simulink model "BMS_V4"  (R2017b)
settings: Solver=FixedStepDiscrete  StartTime=0.0  StopTime=inf  FixedStep=BASETIME  RelTol=1e-3  EnableMultiTasking=on
values from neighbouring files (symbols this model uses):
  AKT_BALANCE = uint16(8)    [BMS_V4_config.m]
  BALANCE = uint16(4)    [BMS_V4_config.m]
  BALANCE_RESISTOR = int32(5)    [BMS_V4_config.m]
  BALANCE_VEC = uint16(8)    [BMS_V4_config.m]
  CELL_SOC = uint16(7)    [BMS_V4_config.m]
  CELL_STATE = uint16(3)    [BMS_V4_config.m]
  CELL_TEMPERATURE = uint16(6)    [BMS_V4_config.m]
  CELL_VOLTAGE = uint16(5)    [BMS_V4_config.m]
  CELLACTBITFIELD = hex2dec('300')    [BMS_V4_config.m]
  CELLDEACTBITFIELD = hex2dec('100')    [BMS_V4_config.m]
  CELLT_BURST = uint16(6)    [BMS_V4_config.m]
  CELLV_BURST = uint16(5)    [BMS_V4_config.m]
  CLK_CYC_timer_1 = 586    [BMS_V4_config.m]
  CLK_CYC_timer_2 = 5860    [BMS_V4_config.m]
  CLK_CYC_timer_3 = 280    [BMS_V4_config.m]
  CLK_CYC_timer_4 = 586*100    (= 58600)    [BMS_V4_config.m]
  CLK_CYC_timer_5 = 5800*2    (= 11600)    [BMS_V4_config.m]
  CLK_CYC_timer_6 = 320    [BMS_V4_config.m]
  CN_CELLS = int32(40*3600)    [BMS_V4_config.m]
  CONTACTOR = uint16(1)    [BMS_V4_config.m]
  CONTACTOR_LOCKED = uint16(0)    [BMS_V4_config.m]
  CONTACTOR_UNLOCKED = uint16(1)    [BMS_V4_config.m]
  DEBUG_SEND_STATES = uint16(hex2dec('01'))    [BMS_V4_config.m]
  DELTA_SOC_BALANCE = int32(5*1e6)    [BMS_V4_config.m]
  DELTA_SOC_BALANCE_OFF = int32(1*1e5)    [BMS_V4_config.m]
  DETERMINE_MODEL_PARAMETER_ACT = uint16(100)    [BMS_V4_config.m]
  DETERMINE_MODEL_PARAMETER_SCC = uint16(101)    [BMS_V4_config.m]
  ERROR = uint16(1)    [BMS_V4_config.m]
  EXTERN_SIGNALS = uint16(1)    [BMS_V4_config.m]
  FREQUENCY_STEPS = uint16([25 50 75 100 150 250 500 750                                      1000 1500 2500 5000 7500                                      10010 10015 10025 10050 10075                                      10100 10150 10250 10500 10750                                      11000 11500])    [BMS_V4_config.m]
  GET_IMAG_PART_MFC = uint16(9)    [BMS_V4_config.m]
  GET_IMAG_PART_MSF = uint16(4)    [BMS_V4_config.m]
  GET_REAL_PART_MFC = uint16(8)    [BMS_V4_config.m]
  GET_REAL_PART_MSF = uint16(3)    [BMS_V4_config.m]
  IMU = uint16(7)    [BMS_V4_config.m]
  IMU_AMP_OFF = uint16(5)    [BMS_V4_config.m]
  IMU_DATA_READ_LOCUS_ACT = uint16(6)    [BMS_V4_config.m]
  IMU_DATA_READ_LOCUS_SCC = uint16(7)    [BMS_V4_config.m]
  IMU_DEBUG = uint16(9)    [BMS_V4_config.m]
  IMU_GET_DATA_MFC = uint16(8)    [BMS_V4_config.m]
  IMU_GET_DATA_MSF = uint16(3)    [BMS_V4_config.m]
  IMU_OFFSET_POLLING = uint16(11)    [BMS_V4_config.m]
  IMU_POLLING = uint16(2)    [BMS_V4_config.m]
  IMU_POWER = uint16(10)    [BMS_V4_config.m]
  IMU_SEND_IMAG = uint16(11)    [BMS_V4_config.m]
  IMU_SEND_REAL = uint16(10)    [BMS_V4_config.m]
  INDEX_IMAGPART = uint16(2)    [BMS_V4_config.m]
  INDEX_REALPART = uint16(1)    [BMS_V4_config.m]
  INFO = uint16(2)    [BMS_V4_config.m]
  INIT_OFFSET_AMPLITUDE = uint16(2)    [BMS_V4_config.m]
  LINE_CURRENT = uint16(3)    [BMS_V4_config.m]
  LINE_CURRENT_CANA = uint16(4)    [BMS_V4_config.m]
  LINE_CURRENT_SWITCH_THRESHOLD = int32(2*1e6)    [BMS_V4_config.m]
  NUM_OF_CELLS = uint16(16)    [BMS_V4_config.m]
  NUM_OF_FREQUENCIES_PSO = uint16(14)    [BMS_V4_config.m]
  NUM_OF_LINES = uint16(1)    [BMS_V4_config.m]
  NUM_OF_PARAMETER = single(5)    [BMS_V4_config.m]
  NUM_OF_SOC_POINTS = uint16(110)    [BMS_V4_config.m]
  P_L_BOUND = single([0.05;0.01;0.1;0.01;0.1])    [BMS_V4_config.m]
  P_U_BOUND = single([0.50;0.20;0.9;0.06;60])    [BMS_V4_config.m]
  PARA_ACT_SEND = uint16(101)    [BMS_V4_config.m]
  PARA_DATA_STORE_ACT = uint16(8)    [BMS_V4_config.m]
  PARA_DATA_STORE_SCC = uint16(9)    [BMS_V4_config.m]
  PARA_SCC_SEND = uint16(102)    [BMS_V4_config.m]
  PARTICLE_INIT = single(create_startparticle(P_L_BOUND,P_U_BOUND,NUM_OF_PARTICLE))    [BMS_V4_config.m]
  POLACT = hex2dec('00000BFF')    [BMS_V4_config.m]
  POLDEACT = hex2dec('000008FF')    [BMS_V4_config.m]
  PSO_PARA_DEBUG = uint16(13)    [BMS_V4_config.m]
  REQUEST_SOC_REF = uint16(1000)    [BMS_V4_config.m]
  SCALE_FACTOR_CH1 = single(0.66666666)    [BMS_V4_config.m]
  SCALE_FACTOR_CH2 = single(0.66666666)    [BMS_V4_config.m]
  SEND_CELL_SOC_ABS = uint16(199)    [BMS_V4_config.m]
  SHUT_DOWN_BALANCE_OFF = uint16(3)    [BMS_V4_config.m]
  SHUT_DOWN_BALANCE_ON = uint16(2)    [BMS_V4_config.m]
  START_IMU_MSL = uint16(3)    [BMS_V4_config.m]
  START_IMU_SCC = uint16(1)    [BMS_V4_config.m]
  SWITCH_IMU_OFF = uint16(2)    [BMS_V4_config.m]
  SWITCH_IMU_ON = uint16(1)    [BMS_V4_config.m]
  SWITCH_IMU_ON_OFF = uint16(4)    [BMS_V4_config.m]
  SYSTEM_DEBUG = uint16(12)    [BMS_V4_config.m]
  TIMEOUT_CANA = uint32(5000)    [BMS_V4_config.m]
  TIMEOUT_GATEWAY = uint32(500)    [BMS_V4_config.m]
  TS_SOC = single(0.010)    [BMS_V4_config.m]
  WARNING = uint16(2)    [BMS_V4_config.m]
libraries: c280xlib x44, c2833xlib x5, simulink x2, c2000lib x1, idelinklib_common x1
(part 5 of 8)

== stateflow chart BMS_V4/MRAM_control ==
  state MRAM_send_command(mram_address,mram_data) [function]
  state Init
    en:
  state store_soc_CC
    state init
      en:
      cellNo_soc_cc=uint16(0);
      lineNo_soc_cc=uint16(0);
    state set_wren
      en:
      //write enable CODE 0x00
      MRAM_send_command(uint32(0),uint32(0));
    state Store_soc_CC
      en:
      mram_request=SOC_CC_STORE;
      MRAM_send_command(MRAM_soc_address(cellNo_soc_cc,SOC_CC_STORE),mram_convert_soc(cell_soc_CC[cellNo_soc_cc][lineNo_soc_cc]));
      // (cellNo_soc_cc,STORE_SOC_CC),MRAM_CONVERT_SOC(SoC_Cells_CC[cellNo_soc_cc],1)));
    state inc
      en:
      cellNo_soc_cc=cellNo_soc_cc+uint16(1);
    store_soc_CC.init -> store_soc_CC.set_wren
    store_soc_CC.set_wren -> store_soc_CC.Store_soc_CC : //after(0.0005,sec)
    (junction 64) -> store_soc_CC.set_wren
    (junction 63) -> (junction 64) [order 1] : [cellNo_soc_cc < NUM_OF_CELLS]
    store_soc_CC.Store_soc_CC -> store_soc_CC.inc : //after(0.01,sec)
        | [mram_value_read == true]
        | {mram_value_read = false;}
    store_soc_CC.inc -> (junction 63) : //after(0.0005,sec)
  state store_soc_ABS
    state init
      en:
      cellNo_soc_abs=uint16(0);
      lineNo_soc_abs=uint16(0);
    state set_wren
      en:
      //write enable CODE 0x00
      MRAM_send_command(uint32(0),uint32(0));
    state Store_soc_CC
      en:
      mram_request=SOC_ABS_STORE;
      MRAM_send_command(MRAM_soc_address(cellNo_soc_abs,SOC_ABS_STORE),mram_convert_soc(cell_soc_ABS));
      // (cellNo_soc_cc,STORE_SOC_CC),MRAM_CONVERT_SOC(SoC_Cells_CC[cellNo_soc_cc],1)));
    state inc
      en:
    store_soc_ABS.init -> store_soc_ABS.set_wren
    store_soc_ABS.set_wren -> store_soc_ABS.Store_soc_CC : //after(0.0005,sec)
    store_soc_ABS.Store_soc_CC -> store_soc_ABS.inc : //after(0.01,sec)
        | [mram_value_read == true]
        | {mram_value_read = false;}
  state read_soc_CC
    state init
      en:
      cellNo_soc_cc=uint16(0);
      lineNo_soc_cc=uint16(0);
    state Store_soc_CC
      en:
      mram_value_read = false;
      mram_request=SOC_CC_READ;
      MRAM_send_command(MRAM_soc_address(cellNo_soc_cc,SOC_CC_READ),uint32(0));
      // (cellNo_soc_cc,STORE_SOC_CC),MRAM_CONVERT_SOC(SoC_Cells_CC[cellNo_soc_cc],1)));
    state inc
      en:
      cell_soc_CC[cellNo_soc_cc][lineNo_soc_cc] = mram_convert_unit32_to_int32(spi_rx_msg);
      cellNo_soc_cc=cellNo_soc_cc+uint16(1);
    read_soc_CC.init -> read_soc_CC.Store_soc_CC
    (junction 83) -> read_soc_CC.Store_soc_CC [order 1] : [cellNo_soc_cc < NUM_OF_CELLS]
    read_soc_CC.Store_soc_CC -> read_soc_CC.inc : [mram_value_read == true]
    read_soc_CC.inc -> (junction 83) : //after(0.0005,sec)
  state read_soc_ABS
    state init
      en:
      cellNo_soc_abs=uint16(0);
      lineNo_soc_abs=uint16(0);
    state Store_soc_CC
      en:
      mram_value_read = false;
      mram_request=SOC_ABS_READ;
      MRAM_send_command(MRAM_soc_address(cellNo_soc_abs,SOC_ABS_READ),uint32(0));
      // (cellNo_soc_cc,STORE_SOC_CC),MRAM_CONVERT_SOC(SoC_Cells_CC[cellNo_soc_cc],1)));
    state inc
      en:
      cell_soc_ABS = mram_convert_unit32_to_int32(spi_rx_msg);
    read_soc_ABS.init -> read_soc_ABS.Store_soc_CC
    read_soc_ABS.Store_soc_CC -> read_soc_ABS.inc : [mram_value_read == true]
  state store_imu_data
    state store_imu_data_actual
      state init
        en:
        cellNo_store_imu=uint16(imu_act_cellno-uint16(1));
        lineNo_store_imu=uint16(0);
        soc_store_imu=imu_act_soc;
        freq_ind_store_imu=uint16(imu_act_freq_index-uint16(1));
        store_realpart = mram_convert_single_to_uint32(imu_act_realpart);
        store_imagpart = mram_convert_single_to_uint32(imu_act_imagpart);
        mram_value_stored = false;
      state set_wren
        en:
        //write enable CODE 0x00
        MRAM_send_command(uint32(0),uint32(0));
      state Store_imu_data_soc
        en:
        //mram_value_stored = false;
        mram_request=IMU_DATA_STORE_SOC_POINT;
        MRAM_send_command(MRAM_soc_address(cellNo_store_imu,IMU_DATA_STORE_SOC_POINT),mram_convert_soc(soc_store_imu));
      state set_wren1
        en:
        //write enable CODE 0x00
        MRAM_send_command(uint32(0),uint32(0));
      state Store_imu_data_realpart
        en:
        mram_request=IMU_DATA_STORE_REAL;
        store_address = MRAM_imu_data_address_actual(cellNo_store_imu,freq_ind_store_imu,IMU_DATA_STORE_REAL);
        MRAM_send_command(store_address,store_realpart);
      state set_wren2
        en:
        //write enable CODE 0x00
        MRAM_send_command(uint32(0),uint32(0));
      state Store_imu_data_imagpart
        en:
        mram_request=IMU_DATA_STORE_IMAG;
        store_address = MRAM_imu_data_address_actual(cellNo_store_imu,freq_ind_store_imu,IMU_DATA_STORE_IMAG);
        MRAM_send_command(store_address,store_imagpart);
      store_imu_data.store_imu_data_actual.init -> store_imu_data.store_imu_data_actual.set_wren
      store_imu_data.store_imu_data_actual.set_wren -> Store_imu_data_soc : [mram_value_stored == true]
          | {mram_value_stored = false;}
      Store_imu_data_soc -> set_wren1 : [mram_value_stored == true]
          | {mram_value_stored = false;}
      set_wren1 -> store_imu_data.store_imu_data_actual.Store_imu_data_realpart : //after(0.0005,sec)
          | [mram_value_stored == true]
          | {mram_value_stored = false;}
      store_imu_data.store_imu_data_actual.Store_imu_data_realpart -> store_imu_data.store_imu_data_actual.set_wren2 : [mram_value_stored == true]
          | {mram_value_stored = false;}
      store_imu_data.store_imu_data_actual.set_wren2 -> store_imu_data.store_imu_data_actual.Store_imu_data_imagpart : //after(0.0005,sec)
          | [mram_value_stored == true]
          | {mram_value_stored = false;}
    state store_imu_data_scc
      state init
        en:
        cellNo_store_imu=uint16(imu_act_cellno-uint16(1));
        lineNo_store_imu=uint16(0);
        //convert soc to 0, 1, 2, ..., 98, 99,100% for mram adress config
        soc_point_store = soc_point_counter;
        freq_ind_store_imu=uint16(imu_act_freq_index-uint16(1));
        store_realpart = mram_convert_single_to_uint32(imu_act_realpart);
        store_imagpart = mram_convert_single_to_uint32(imu_act_imagpart);
        mram_value_stored = false;
      state set_wren
        en:
        //write enable CODE 0x00
        MRAM_send_command(uint32(0),uint32(0));
      state Store_imu_data_realpart
        en:
        //mram_value_stored = false;
        mram_request=IMU_DATA_STORE_REAL;
        store_address = MRAM_imu_data_address(cellNo_store_imu,soc_point_store,freq_ind_store_imu,IMU_DATA_STORE_REAL);
        MRAM_send_command(store_address,store_realpart);
      state set_wren2
        en:
        //write enable CODE 0x00
        MRAM_send_command(uint32(0),uint32(0));
      state Store_imu_data_imagpart
        en:
        mram_request=IMU_DATA_STORE_IMAG;
        store_address = MRAM_imu_data_address(cellNo_store_imu,soc_point_store,freq_ind_store_imu,IMU_DATA_STORE_IMAG);
        MRAM_send_command(store_address,store_imagpart);
      store_imu_data.store_imu_data_scc.init -> store_imu_data.store_imu_data_scc.set_wren
      store_imu_data.store_imu_data_scc.set_wren -> store_imu_data.store_imu_data_scc.Store_imu_data_realpart : [mram_value_stored == true]
          | {mram_value_stored = false;}
      store_imu_data.store_imu_data_scc.Store_imu_data_realpart -> store_imu_data.store_imu_data_scc.set_wren2 : [mram_value_stored == true]
          | {mram_value_stored = false;}
      store_imu_data.store_imu_data_scc.set_wren2 -> store_imu_data.store_imu_data_scc.Store_imu_data_imagpart : [mram_value_stored == true]
          | {mram_value_stored = false;}
    (junction 230) -> store_imu_data.store_imu_data_scc.init [order 1] : [imu_function == START_IMU_SCC]
    (junction 230) -> store_imu_data.store_imu_data_actual.init [order 2] : [ imu_function == START_IMU_MSL ]
    store_imu_data.store_imu_data_scc.Store_imu_data_imagpart -> (junction 236) : [mram_value_stored == true]
        | {mram_value_stored = false;}
    store_imu_data.store_imu_data_actual.Store_imu_data_imagpart -> (junction 236) : [mram_value_stored == true]
        | {mram_value_stored = false;}
  state read_imu_data_act
    state read_soc_point_imu_data
      en:
      cellNo_read_locus=mram_cellno_to_read-uint16(1);
      mram_request=IMU_DATA_READ_SOC_POINT;
      MRAM_send_command(MRAM_soc_address(cellNo_read_locus,IMU_DATA_READ_SOC_POINT),uint32(0));
    state store_soc_point_imu_data
      en:
      soc_of_one_locus_act = mram_convert_unit32_to_int32(spi_rx_msg);
      freq_ind_read_locus=uint16(0);
    state read_realpart_imu_data
      en:
      mram_request=IMU_DATA_READ_REAL;
      MRAM_send_command(MRAM_imu_data_address_actual(cellNo_read_locus,freq_ind_read_locus,IMU_DATA_READ_REAL),uint32(0));
    state store_real_part_and_read_imagpart_imu_data
      en:
      one_locus_act[freq_ind_read_locus][uint16(0)] = mram_convert_uint32_to_single(spi_rx_msg);
      mram_request=IMU_DATA_READ_IMAG;
      MRAM_send_command(MRAM_imu_data_address_actual(cellNo_read_locus,freq_ind_read_locus,IMU_DATA_READ_IMAG),uint32(0));
    state store_imag_part
      en:
      one_locus_act[freq_ind_read_locus][uint16(1)] = mram_convert_uint32_to_single(spi_rx_msg);
    read_soc_point_imu_data -> read_imu_data_act.store_soc_point_imu_data : //after(0.01,sec)
        | [mram_value_read == true]
        | {mram_value_read = false;}
    read_imu_data_act.store_soc_point_imu_data -> read_imu_data_act.read_realpart_imu_data : //after(0.01,sec)
        | //[mram_value_read == true]
        | //{mram_value_read = false;}
    (junction 894) -> read_imu_data_act.read_realpart_imu_data
    (junction 893) -> (junction 894)
    read_imu_data_act.read_realpart_imu_data -> store_real_part_and_read_imagpart_imu_data : //after(0.01,sec)
        | [mram_value_read == true]
        | {mram_value_read = false;}
    store_real_part_and_read_imagpart_imu_data -> read_imu_data_act.store_imag_part : //after(0.01,sec)
        | [mram_value_read == true]
        | {mram_value_read = false;}
    read_imu_data_act.store_imag_part -> (junction 893) [order 1] : [freq_ind_read_locus < (NUM_OF_FREQUENCIES-uint16(1))]
        | {freq_ind_read_locus++;}
  state read_imu_data_scc
    state init
      en:
      cellNo_read_locus = mram_cellno_to_read-uint16(1);
      socpoint_read_locus = mram_soc_point_to_read - uint16(1);
      freq_ind_read_locus=uint16(0);
    state read_realpart_imu_data
      en:
      mram_request=IMU_DATA_READ_REAL;
      MRAM_send_command(MRAM_imu_data_address(cellNo_read_locus,socpoint_read_locus,freq_ind_read_locus,IMU_DATA_READ_REAL),uint32(0));
    state store_real_part_and_read_imagpart_imu_data1
      en:
      one_locus_scc[freq_ind_read_locus][uint16(0)] = mram_convert_uint32_to_single(spi_rx_msg);
      mram_request=IMU_DATA_READ_IMAG;
      MRAM_send_command(MRAM_imu_data_address(cellNo_read_locus,socpoint_read_locus,freq_ind_read_locus,IMU_DATA_READ_IMAG),uint32(0));
    state store_imag_part
      en:
      one_locus_scc[freq_ind_read_locus][uint16(1)] = mram_convert_uint32_to_single(spi_rx_msg);
    read_imu_data_scc.init -> read_imu_data_scc.read_realpart_imu_data : after(0.0005,sec)
    (junction 871) -> read_imu_data_scc.read_realpart_imu_data
    (junction 875) -> (junction 871)
    read_imu_data_scc.read_realpart_imu_data -> store_real_part_and_read_imagpart_imu_data1 : //after(0.01,sec)
        | [mram_value_read == true]
        | {mram_value_read = false;}
    store_real_part_and_read_imagpart_imu_data1 -> read_imu_data_scc.store_imag_part : //after(0.01,sec)
        | [mram_value_read == true]
        | {mram_value_read = false;}
    read_imu_data_scc.store_imag_part -> (junction 875) [order 1] : [freq_ind_read_locus < (NUM_OF_FREQUENCIES-uint16(1))]
        | {freq_ind_read_locus++;}
  state store_para_data_act
    //stores all 6 parameter
    // of one cell
    state init
      en:
      num_para_store = uint16(0);
      cellNo_store_para=uint16(para_act_cellno-uint16(1));
      lineNo_store_para=uint16(0);
    state select_parameter
      en:
      store_parameter = mram_convert_single_to_uint32(parameter_one_cell_act[num_para_store]);
    state set_wren
      en:
      //write enable CODE 0x00
      MRAM_send_command(uint32(0),uint32(0));
    state Store_para_data
      en:
      //mram_value_stored = false;
      mram_request=PARA_STORE_ACT;
      store_address = MRAM_para_address_act(cellNo_store_para,num_para_store, PARA_STORE_ACT);
      MRAM_send_command(store_address,store_parameter);
    store_para_data_act.init -> store_para_data_act.select_parameter
    (junction 659) -> store_para_data_act.select_parameter
    (junction 657) -> (junction 659) [order 1] : [num_para_store < NUM_OF_PARAMETER]
        | {num_para_store++;}
        | // num of parameter = 5, but here we save 6 parameter
        | // parameter 6 is L2norm
    store_para_data_act.select_parameter -> store_para_data_act.set_wren
    (junction 745) -> (junction 746)
    store_para_data_act.set_wren -> store_para_data_act.Store_para_data : [mram_value_stored == true]
        | {mram_value_stored = false;}
    store_para_data_act.Store_para_data -> (junction 657) : [mram_value_stored == true]
        | {mram_value_stored = false;}
    (junction 657) -> (junction 744) [order 2]
    (junction 744) -> (junction 745)
  state store_para_data_scc
    //stores all  parameter of scc  0% SoC -> 100%SoC
    //of one cell
    state init
      en:
      num_para_store = uint16(0);
      cellNo_store_para = para_act_cellno-uint16(1);
      lineNo_store_para = uint16(0);
      soc_point_store_scc = uint16(0); // 0 indexing in simulink 1-101 for 0% - 100%
    state select_parameter
      en:
      store_parameter = mram_convert_single_to_uint32(parameter_one_cell_scc[soc_point_store_scc][num_para_store]);
      store_address = MRAM_para_address_scc(cellNo_store_para,num_para_store,soc_point_store_scc, PARA_STORE_SCC);
    state set_wren
      en:
      //write enable CODE 0x00
      MRAM_send_command(uint32(0),uint32(0));
    state Store_para_data
      en:
      //mram_value_stored = false;
      mram_request=PARA_STORE_SCC;
      MRAM_send_command(store_address,store_parameter);
    store_para_data_scc.init -> store_para_data_scc.select_parameter
    (junction 924) -> store_para_data_scc.select_parameter [order 1] : //[soc_point_store_scc < (NUM_OF_SOC_POINTS-uint16(1))]
        | [soc_point_store_scc < (last_soc_point_index - uint16(1))]
        | {soc_point_store_scc ++;}
    (junction 912) -> (junction 924)
    (junction 923) -> store_para_data_scc.select_parameter
    (junction 926) -> (junction 923) [order 1] : [num_para_store < NUM_OF_PARAMETER]
        | {num_para_store++;}
        | // num of parameter = 5, but here we save 6 parameter
        | // parameter 6 is L2norm
    store_para_data_scc.select_parameter -> store_para_data_scc.set_wren
    store_para_data_scc.set_wren -> store_para_data_scc.Store_para_data : [mram_value_stored == true]
        | {mram_value_stored = false;}
    store_para_data_scc.Store_para_data -> (junction 926) : [mram_value_stored == true]
        | {mram_value_stored = false;}
    (junction 926) -> (junction 925) [order 2] : {num_para_store = uint16(0);}
    (junction 925) -> (junction 912)
  state read_para_data_act
    // read parameter set from last impedance measurement of one cell.
    // global variable parameterset_one_cell coresponding soc is stored at soc adress from actual imu
    state read_soc_point_para_data
      en:
      num_para_read = uint16(0);
      cellNo_read_para=para_act_cellno-uint16(1);
      mram_request=IMU_DATA_READ_SOC_POINT;
      MRAM_send_command(MRAM_soc_address(cellNo_read_para,IMU_DATA_READ_SOC_POINT),uint32(0));
    state store_soc_point_imu_data
      en:
      soc_of_one_para_act = mram_convert_unit32_to_int32(spi_rx_msg); // same soc of locus meas act
      //soc_of_one_locus_act = mram_convert_unit32_to_int32(spi_rx_msg);
    state Read_para_data
      en:
      //mram_value_stored = false;
      mram_request=PARA_READ_ACT;
      MRAM_send_command(MRAM_para_address_act(cellNo_read_para,num_para_read, PARA_READ_ACT),uint32(0));
    state save_para_data
      en:
      parameter_one_cell_act[num_para_read] = mram_convert_uint32_to_single(spi_rx_msg);
    read_soc_point_para_data -> read_para_data_act.store_soc_point_imu_data : //after(0.01,sec)
        | [mram_value_read == true]
        | {mram_value_read = false;}
    read_para_data_act.store_soc_point_imu_data -> read_para_data_act.Read_para_data : //after(0.01,sec)
        | //[mram_value_read == true]
        | //{mram_value_read = false;}
    (junction 1036) -> read_para_data_act.Read_para_data
    (junction 1029) -> (junction 1036) [order 1] : [num_para_read < NUM_OF_PARAMETER]
        | {num_para_read++;}
        | // num of parameter = 5, but here we save 6 parameter
        | // parameter 6 is L2norm
    read_para_data_act.Read_para_data -> read_para_data_act.save_para_data : //after(0.01,sec)
        | [mram_value_read == true]
        | {mram_value_read = false;}
    (junction 1031) -> (junction 1035)
    read_para_data_act.save_para_data -> (junction 1029)
    (junction 1029) -> (junction 1030) [order 2]
    (junction 1030) -> (junction 1031)
  state read_para_data_scc
    // read parameter set from last impedance measurement of one cell.
    // global variable parameterset_one_cell coresponding soc is stored at soc adress from actual imu
    state init
      en:
      num_para_read = uint16(0);
      cellNo_read_para=para_act_cellno-uint16(1);
      soc_point_read_scc = uint16(0); // 0 indexing in simulink 1-101 for 0% - 100%
    state Read_para_data
      en:
      //mram_value_stored = false;
      mram_request=PARA_READ_SCC;
      MRAM_send_command(MRAM_para_address_scc(cellNo_read_para,num_para_read,soc_point_read_scc, PARA_READ_SCC),uint32(0));
    state save_para_data
      en:
      parameter_one_cell_scc[soc_point_read_scc][num_para_read] = mram_convert_uint32_to_single(spi_rx_msg);
    read_para_data_scc.init -> read_para_data_scc.Read_para_data
    (junction 1042) -> read_para_data_scc.Read_para_data [order 1] : //[soc_point_read_scc < (NUM_OF_SOC_POINTS-uint16(1))]
        | [soc_point_read_scc < (last_soc_point_index - uint16(1))]
        | {soc_point_read_scc ++;}
    (junction 1041) -> read_para_data_scc.Read_para_data
    (junction 1044) -> (junction 1042)
    (junction 1043) -> (junction 1041) [order 1] : [num_para_read < NUM_OF_PARAMETER]
        | {num_para_read++;}
        | // num of parameter = 5, but here we save 6 parameter
        | // parameter 6 is L2norm
    read_para_data_scc.Read_para_data -> read_para_data_scc.save_para_data : //after(0.01,sec)
        | [mram_value_read == true]
        | {mram_value_read = false;}
    read_para_data_scc.save_para_data -> (junction 1043) : //after(0.01,sec)
    (junction 1043) -> (junction 1045) [order 2] : {num_para_read = uint16(0);}
    (junction 1045) -> (junction 1044)
  state store_soc_SCC
    state init
      en:
      soc_point_scc = uint16(0);
    state set_wren
      en:
      //write enable CODE 0x00
      MRAM_send_command(uint32(0),uint32(0));
    state Store_soc_SCC
      en:
      mram_request=SOC_SCC_STORE;
      MRAM_send_command(MRAM_soc_scc_address(soc_point_scc,SOC_SCC_STORE),mram_convert_soc(soc_points_of_scc[soc_point_scc]));
      // (cellNo_soc_cc,STORE_SOC_CC),MRAM_CONVERT_SOC(SoC_Cells_CC[cellNo_soc_cc],1)));
    state inc
      en:
      soc_point_scc=soc_point_scc+uint16(1);
    store_soc_SCC.init -> store_soc_SCC.set_wren
    store_soc_SCC.set_wren -> Store_soc_SCC : //after(0.0005,sec)
    (junction 943) -> store_soc_SCC.set_wren
    (junction 944) -> (junction 943) [order 1] : //[soc_point_scc < NUM_OF_SOC_POINTS]
        | [soc_point_scc < last_soc_point_index]
    Store_soc_SCC -> store_soc_SCC.inc : //after(0.01,sec)
        | [mram_value_read == true]
        | {mram_value_read = false;}
    store_soc_SCC.inc -> (junction 944) : //after(0.0005,sec)
  state read_soc_SCC
    state init
      en:
      soc_point_scc = uint16(0);
    state set_wren
      en:
      //write enable CODE 0x00
      MRAM_send_command(uint32(0),uint32(0));
    state Read_soc_SCC
      en:
      mram_request=SOC_SCC_READ;
      MRAM_send_command(MRAM_soc_scc_address(soc_point_scc,SOC_SCC_READ),uint32(0));
    state store_value_and_inc
      en:
      soc_points_of_scc[soc_point_scc] = mram_convert_unit32_to_int32(spi_rx_msg);
      soc_point_scc=soc_point_scc+uint16(1);
    read_soc_SCC.init -> read_soc_SCC.set_wren
    read_soc_SCC.set_wren -> Read_soc_SCC : //after(0.0005,sec)
    (junction 974) -> read_soc_SCC.set_wren
    (junction 975) -> (junction 974) [order 1] : //[soc_point_scc < NUM_OF_SOC_POINTS]
        | [soc_point_scc < last_soc_point_index]
    Read_soc_SCC -> store_value_and_inc : //after(0.01,sec)
        | [mram_value_read == true]
        | {mram_value_read = false;}
    store_value_and_inc -> (junction 975) : //after(0.0005,sec)
  state store_last_soc_index
    state set_wren
      en:
      //write enable CODE 0x00
      MRAM_send_command(uint32(0),uint32(0));
    state Store_soc_CC
      en:
      MRAM_send_command(MRAM_address_scc_soc_index(STORE_LAST_SOC_INDEX),uint32(last_soc_point_index));
    state wait_
      en:
    store_last_soc_index.set_wren -> store_last_soc_index.Store_soc_CC : //after(0.0005,sec)
    store_last_soc_index.Store_soc_CC -> wait_ : //after(0.01,sec)
        | [mram_value_read == true]
        | {mram_value_read = false;}
  state read_last_soc_index
    state Store_soc_CC
      en:
      MRAM_send_command(MRAM_address_scc_soc_index(READ_LAST_SOC_INDEX),uint32(0));
    state save
      en:
      last_soc_point_index = uint16(spi_rx_msg);
    read_last_soc_index.Store_soc_CC -> save : //after(0.01,sec)
        | [mram_value_read == true]
        | {mram_value_read = false;}
  (junction 1090) -> store_last_soc_index.set_wren [order 1] : [ mram_command...
      | [STORE_LAST_SOC_INDEX_SCC - uint16(1)]...
      |  == true ]
  (junction 1111) -> read_last_soc_index.Store_soc_CC : [ mram_command...
      | [READ_LAST_SOC_INDEX_SCC - uint16(1)]...
      |  == true ]
  (junction 1035) -> (junction 560) : {mram_command...
      | [PARA_DATA_READ_ACT-uint16(1)]...
      | = false;}
  (junction 1042) -> (junction 638) [order 2] : {mram_command...
      | [PARA_DATA_READ_SCC-uint16(1)]...
      | = false;}
  (junction 989) -> read_soc_SCC.init [order 1] : [ mram_command...
      | [SOC_SCC_READ - uint16(1)]...
      |  == true ]
  (junction 958) -> store_soc_SCC.init [order 1] : [ mram_command...
      | [SOC_SCC_STORE - uint16(1)]...
      |  == true ]
  read_imu_data_scc.store_imag_part -> (junction 851) [order 2] : {mram_command...
      | [IMU_DATA_READ_LOCUS_SCC-uint16(1)]...
      | = false;}
  read_imu_data_act.store_imag_part -> (junction 178) [order 2] : {mram_command...
      | [IMU_DATA_READ_LOCUS_ACT-uint16(1)]...
      | = false;}
  (junction 849) -> read_imu_data_scc.init [order 1] : [ mram_command...
      | [IMU_DATA_READ_LOCUS_SCC-uint16(1)]...
      |  == true ]
  (junction 746) -> (junction 451) : {mram_command...
      | [PARA_DATA_STORE_ACT-uint16(1)]...
      | = false;}
  (junction 63) -> (junction 31) [order 2] : {mram_command...
      | [SOC_CC_STORE-uint16(1)]...
      | = false;}
  (junction 83) -> (junction 100) [order 2] : {mram_command...
      | [SOC_CC_READ-uint16(1)]...
      | = false;}
  (junction 21) -> store_soc_ABS.init [order 1] : [ mram_command...
      | [SOC_ABS_STORE-uint16(1)] ...
      | ==true ]
  (junction 728) -> read_soc_ABS.init [order 1] : [ mram_command...
      | [SOC_ABS_READ-uint16(1)]...
      |  == true ]
  read_soc_ABS.inc -> (junction 730) : {mram_command...
      | [SOC_ABS_READ-uint16(1)]...
      | = false;}
  (junction 975) -> (junction 990) [order 2] : {mram_command...
      | [SOC_SCC_READ-uint16(1)]...
      | = false;}
  (junction 944) -> (junction 962) [order 2] : {mram_command...
      | [SOC_SCC_STORE-uint16(1)]...
      | = false;}
  wait_ -> (junction 1094) : {mram_command...
      | [STORE_LAST_SOC_INDEX_SCC-uint16(1)]...
      | = false;}
  save -> (junction 1115) : {mram_command...
      | [READ_LAST_SOC_INDEX_SCC-uint16(1)]...
      | = false;}
  (junction 181) -> read_soc_point_imu_data [order 1] : [ mram_command...
      | [IMU_DATA_READ_LOCUS_ACT-uint16(1)]...
      |  == true ]
  (default) -> Init
  Init -> (junction 4) : [ (mram_command[0] || ...
      |    mram_command[1] || ...
      |    mram_command[2] || ...
      |    mram_command[3] || ...
      |    mram_command[4] || ...
      |    mram_command[5] || ...
      |    mram_command[6] || ...
      |    mram_command[7] || ...
      |    mram_command[8] || ...
      |    mram_command[9] || ...
      |    mram_command[10] || ...
      |    mram_command[11] || ...
      |    mram_command[12] || ...
      |    mram_command[13] || ...
      |    mram_command[14]) != 0]
  (junction 4) -> (junction 19)
  (junction 31) -> Init
  (junction 924) -> (junction 631) [order 2] : {mram_command...
      | [PARA_DATA_STORE_SCC-uint16(1)]...
      | = false;}
  (junction 236) -> (junction 120) : {mram_command...
      | [IMU_DATA_STORE-uint16(1)]...
      | = false;}
  (junction 19) -> store_soc_CC.init [order 1] : [ mram_command...
      | [SOC_CC_STORE-uint16(1)]...
      |  == true ]
  (junction 33) -> (junction 31)
  (junction 19) -> (junction 21) [order 2]
  store_soc_ABS.inc -> (junction 33) : {mram_command...
      | [SOC_ABS_STORE-uint16(1)]...
      | = false;}
  (junction 100) -> (junction 33)
  (junction 21) -> (junction 97) [order 2]
  (junction 730) -> (junction 100)
  (junction 97) -> (junction 728) [order 2]
  (junction 97) -> read_soc_CC.init [order 1] : [ mram_command...
      | [SOC_CC_READ-uint16(1)]...
      |  == true ]
  (junction 120) -> (junction 730)
  (junction 728) -> (junction 123) [order 2]
  (junction 123) -> (junction 230) [order 1] : [ mram_command...
      | [IMU_DATA_STORE-uint16(1)]...
      |  == true ]
  (junction 178) -> (junction 120)
  (junction 123) -> (junction 181) [order 2]
  (junction 181) -> (junction 849) [order 2]
  (junction 851) -> (junction 178)
  (junction 451) -> (junction 851)
  (junction 849) -> (junction 452) [order 2]
  (junction 452) -> store_para_data_act.init [order 1] : [ mram_command...
      | [PARA_DATA_STORE_ACT-uint16(1)]...
      |  == true ]
  (junction 631) -> (junction 451)
  (junction 452) -> (junction 628) [order 2]
  (junction 628) -> store_para_data_scc.init [order 2] : [ mram_command...
      | [PARA_DATA_STORE_SCC-uint16(1)]...
      |  == true ]
  (junction 628) -> (junction 561) [order 1]
  (junction 560) -> (junction 631)
  (junction 561) -> read_soc_point_para_data [order 2] : [ mram_command...
      | [PARA_DATA_READ_ACT-uint16(1)]...
      |  == true ]
  (junction 638) -> (junction 560)
  (junction 561) -> (junction 637) [order 1]
  (junction 637) -> read_para_data_scc.init [order 1] : [ mram_command...
      | [PARA_DATA_READ_SCC-uint16(1)]...
      |  == true ]
  (junction 962) -> (junction 638)
  (junction 637) -> (junction 958) [order 2]
  (junction 990) -> (junction 962)
  (junction 958) -> (junction 989) [order 2]
  (junction 1094) -> (junction 990)
  (junction 989) -> (junction 1090) [order 2]
  (junction 1115) -> (junction 1094)
  (junction 1090) -> (junction 1111) [order 2]
  data: mram_address function_input uint32; mram_data function_input uint32; soc_point function_input uint16; CODE_SOC function_input uint16; mram_address function_output uint32; cell_no function_input uint16; CODE_SOC function_input uint16; mram_address function_output uint32; cell_no function_input uint16; soc_point function_input uint16; mram_address function_output uint32; freq_ind function_input uint16; CODE_IMU_DATA function_input uint16; cell_no function_input uint16; mram_address function_output uint32; freq_ind function_input uint16; CODE_IMU_DATA function_input uint16; cell_no function_input uint16; para_num function_input double; CODE_PARA function_input uint16; mram_address function_output uint32; CODE_INDEX function_input uint16; mram_address function_output uint32; cell_no function_input uint16; para_num function_input double; soc_point function_input double; CODE_PARA function_input uint16; mram_address function_output uint32; value function_input uint32; value_converted function_output single; value function_input single; value_converted function_output uint32; value function_input uint32; value_converted function_output int32; act_soc function_input int32; value function_output uint32; mram_command data_store_memory; SOC_CC_STORE parameter; SOC_CC_READ parameter; SOC_ABS_STORE parameter; SOC_ABS_READ parameter; IMU_DATA_STORE parameter; BASIS_ADDRESS_SOC parameter; mram_value_stored data_store_memory; mram_request data_store_memory; cell_soc_CC data_store_memory; cellNo_soc_cc local uint16; lineNo_soc_cc local uint16; NUM_OF_CELLS parameter; mram_value_read data_store_memory; BASIS_ADDRESS_LOCUS parameter; IMU_DATA_STORE_REAL parameter; IMU_DATA_STORE_IMAG parameter; NUM_OF_SOC_POINTS parameter; NUM_OF_FREQUENCIES parameter; imu_act_cellno data_store_memory; imu_act_lineno data_store_memory; imu_act_freq_index data_store_memory; imu_act_realpart data_store_memory; imu_act_imagpart data_store_memory; IMU_DATA_READ_IMAG parameter; IMU_DATA_READ_REAL parameter; mram_soc_point_to_read data_store_memory; mram_cellno_to_read data_store_memory; freq_ind_read_locus local uint16; IMU_DATA_READ_LOCUS_SCC parameter; IMU_DATA_READ_LOCUS_ACT parameter; BASIS_ADDRESS_LOCUS_SCC parameter; IMU_DATA_STORE_SOC_POINT parameter; IMU_DATA_READ_SOC_POINT parameter; imu_function data_store_memory; START_IMU_SCC parameter; spi_rx_msg data_store_memory; imu_act_soc data_store_memory; freq_ind_store_imu local uint16; cellNo_store_imu local uint16; lineNo_store_imu local uint16; soc_store_imu local int32; cellNo_read_locus local uint16; START_IMU_MSL parameter; store_address local uint32; store_imagpart local uint32; store_realpart local uint32; test local uint32; test2 local uint32 =1000; soc_point_store local uint16; soc_point_counter data_store_memory; BASIS_ADDRESS_PARA_SCC parameter; BASIS_ADDRESS_PARA_ACT parameter; BASIS_ADDRESS_STATUS parameter; PARA_DATA_STORE_ACT parameter; PARA_DATA_READ_ACT parameter; parameter_one_cell_act data_store_memory; PARA_DATA_READ_SCC parameter; PARA_DATA_STORE_SCC parameter; PARA_STORE_ACT parameter; PARA_STORE_SCC parameter; PARA_READ_ACT parameter; PARA_READ_SCC parameter; para_act_cellno data_store_memory; lineNo_store_para local uint16; cellNo_store_para local uint16; num_para_store local uint16; store_parameter local uint32; NUM_OF_PARAMETER parameter; cell_soc_ABS data_store_memory; cellNo_soc_abs local uint16; lineNo_soc_abs local uint16; one_locus_act data_store_memory; one_locus_scc data_store_memory; soc_of_one_locus_act data_store_memory; parameter_one_cell_scc data_store_memory; socpoint_read_locus local uint16; soc_point_store_scc local uint16; SOC_SCC_STORE parameter; SOC_SCC_READ parameter; soc_points_of_scc data_store_memory; BASIS_ADDRESS_SOC_SCC parameter; soc_point_scc local uint16; soc_of_one_para_act data_store_memory; num_para_read local uint16; cellNo_read_para local uint16; soc_point_read_scc local uint16; last_soc_point_index data_store_memory; STORE_LAST_SOC_INDEX_SCC parameter; READ_LAST_SOC_INDEX_SCC parameter; READ_LAST_SOC_INDEX parameter; STORE_LAST_SOC_INDEX parameter; ADDRESS_LAST_SOC_INDEX parameter
  events: trigger_MRAM input FUNCTION_CALL_EVENT
  function mram_address =MRAM_soc_scc_address(soc_point,CODE_SOC):
    | function mram_address =MRAM_soc_scc_address(soc_point,CODE_SOC)
    | 
    | CODE = uint16([0 0 0 0]);
    | 
    | address_single=single(0);
    | 
    | if CODE_SOC == SOC_SCC_STORE
    |     CODE = uint16([hex2dec('02') 0 0 0]);
    |     address_single=single(soc_point)*4+single(BASIS_ADDRESS_SOC_SCC);
    | end
    | 
    | if CODE_SOC == SOC_SCC_READ
    |     CODE = uint16([hex2dec('03') 0 0 0]);
    |     address_single=single(soc_point)*4+single(BASIS_ADDRESS_SOC_SCC);
    | end
    | 
    | %address=typecast(address_single,'uint32');
    | address = uint32(address_single);
    | 
    | % änderung reihenfolge um adresse richtig für maram zu versenden
    | CODE(4)= uint16(bitand(uint32(hex2dec('000000ff')),address));
    | CODE(3)= uint16(bitand(uint32(hex2dec('000000ff')),bitshift(address,-8)));
    | CODE(2)= uint16(bitand(uint32(hex2dec('000000ff')),bitshift(address,-16)));
    | 
    | 
    | x1=uint16(bitand(uint16(hex2dec('00ff')),uint16(CODE(1))));
    | x2=uint16(bitand(uint16(hex2dec('ff00')),uint16(bitshift(uint16(CODE(2)),8))));
    | x3=uint16(bitand(uint16(hex2dec('00ff')),uint16(CODE(3))));
    | x4=uint16(bitand(uint16(hex2dec('ff00')),uint16(bitshift(uint16(CODE(4)),8))));
    | 
    | x11=uint16(bitor(x1,x2));
    | x12=uint16(bitor(x3,x4));
    | 
    | mram_address=uint32(bitor(uint32(x11),bitshift(uint32(x12),16)));
    | 
    | end
  function mram_address =MRAM_soc_address(cell_no,CODE_SOC):
    | function mram_address =MRAM_soc_address(cell_no,CODE_SOC)
    | 
    | CODE = uint16([0 0 0 0]);
    | 
    | address_single=single(0);
    | 
    | if CODE_SOC == SOC_CC_STORE
    |     CODE = uint16([hex2dec('02') 0 0 0]);
    |     address_single=single(cell_no)*12+single(BASIS_ADDRESS_SOC);
    | end
    | if CODE_SOC == SOC_ABS_STORE
    |     CODE = uint16([hex2dec('02') 0 0 0]);
    |     address_single=single(cell_no)*12+4+single(BASIS_ADDRESS_SOC);
    | end
    | if CODE_SOC == IMU_DATA_STORE_SOC_POINT
    |     CODE = uint16([hex2dec('02') 0 0 0]);
    |     address_single=single(cell_no)*12+8+single(BASIS_ADDRESS_SOC);    
    | end
    | 
    | if CODE_SOC == SOC_CC_READ
    |     CODE = uint16([hex2dec('03') 0 0 0]);
    |     address_single=single(cell_no)*12+single(BASIS_ADDRESS_SOC);
    | end
    | if CODE_SOC == SOC_ABS_READ
    |     CODE = uint16([hex2dec('03') 0 0 0]);
    |     address_single=single(cell_no)*12+4+single(BASIS_ADDRESS_SOC);
    | end
    | if CODE_SOC == IMU_DATA_READ_SOC_POINT
    |     CODE = uint16([hex2dec('03') 0 0 0]);
    |     address_single=single(cell_no)*12+8+single(BASIS_ADDRESS_SOC);    
    | end
    | 
    | %address=typecast(address_single,'uint32');
    | address = uint32(address_single);
    | 
    | % änderung reihenfolge um adresse richtig für maram zu versenden
    | CODE(4)= uint16(bitand(uint32(hex2dec('000000ff')),address));
    | CODE(3)= uint16(bitand(uint32(hex2dec('000000ff')),bitshift(address,-8)));
    | CODE(2)= uint16(bitand(uint32(hex2dec('000000ff')),bitshift(address,-16)));
    | 
    | 
    | x1=uint16(bitand(uint16(hex2dec('00ff')),uint16(CODE(1))));
    | x2=uint16(bitand(uint16(hex2dec('ff00')),uint16(bitshift(uint16(CODE(2)),8))));
    | x3=uint16(bitand(uint16(hex2dec('00ff')),uint16(CODE(3))));
    | x4=uint16(bitand(uint16(hex2dec('ff00')),uint16(bitshift(uint16(CODE(4)),8))));
    | 
    | x11=uint16(bitor(x1,x2));
    | x12=uint16(bitor(x3,x4));
    | 
    | mram_address=uint32(bitor(uint32(x11),bitshift(uint32(x12),16)));
    | 
    | end
  function mram_address =MRAM_imu_data_address(cell_no,soc_point,freq_ind,...:
    | function mram_address =MRAM_imu_data_address(cell_no,soc_point,freq_ind,...
    | CODE_IMU_DATA)
    | 
    | CODE = uint16([0 0 0 0]);
    | 
    | address_single=single(0);
    | 
    | if CODE_IMU_DATA == IMU_DATA_STORE_REAL
    |     CODE = uint16([hex2dec('02') 0 0 0]);
    |     address_single=(single(cell_no)*(single(NUM_OF_FREQUENCIES)*8)...
    |         *single(NUM_OF_SOC_POINTS))+...
    |         (single(soc_point)*single(NUM_OF_FREQUENCIES)*8)+...
    |         (single(freq_ind)*8)+single(BASIS_ADDRESS_LOCUS_SCC);
    | end
    | if CODE_IMU_DATA == IMU_DATA_STORE_IMAG
    |     CODE = uint16([hex2dec('02') 0 0 0]);
    |     address_single=(single(cell_no)*(single(NUM_OF_FREQUENCIES)*8)...
    |         *single(NUM_OF_SOC_POINTS))+...
    |         (single(soc_point)*single(NUM_OF_FREQUENCIES)*8)+...
    |         (single(freq_ind)*8)+4+single(BASIS_ADDRESS_LOCUS_SCC);
    | end
    | if CODE_IMU_DATA == IMU_DATA_READ_REAL
    |     CODE = uint16([hex2dec('03') 0 0 0]);
    |    address_single=(single(cell_no)*(single(NUM_OF_FREQUENCIES)*8)...
    |         *single(NUM_OF_SOC_POINTS))+...
    |         (single(soc_point)*single(NUM_OF_FREQUENCIES)*8)+...
    |         (single(freq_ind)*8)+single(BASIS_ADDRESS_LOCUS_SCC);
    | end
    | if CODE_IMU_DATA == IMU_DATA_READ_IMAG
    |     CODE = uint16([hex2dec('03') 0 0 0]);
    |     address_single=(single(cell_no)*(single(NUM_OF_FREQUENCIES)*8)...
    |         *single(NUM_OF_SOC_POINTS))+...
    |         (single(soc_point)*single(NUM_OF_FREQUENCIES)*8)+...
    |         (single(freq_ind)*8)+4+single(BASIS_ADDRESS_LOCUS_SCC);
    | end
    | 
    | 
    | %address=typecast(address_single,'uint32');
    | address = uint32(address_single);
    | 
    | % änderung reihenfolge um adresse richtig für maram zu versenden
    | CODE(4)= uint16(bitand(uint32(hex2dec('000000ff')),address));
    | CODE(3)= uint16(bitand(uint32(hex2dec('000000ff')),bitshift(address,-8)));
    | CODE(2)= uint16(bitand(uint32(hex2dec('000000ff')),bitshift(address,-16)));
    | 
    | 
    | x1=uint16(bitand(uint16(hex2dec('00ff')),uint16(CODE(1))));
    | x2=uint16(bitand(uint16(hex2dec('ff00')),uint16(bitshift(uint16(CODE(2)),8))));
    | x3=uint16(bitand(uint16(hex2dec('00ff')),uint16(CODE(3))));
    | x4=uint16(bitand(uint16(hex2dec('ff00')),uint16(bitshift(uint16(CODE(4)),8))));
    | 
    | x11=uint16(bitor(x1,x2));
    | x12=uint16(bitor(x3,x4));
    | 
    | mram_address=uint32(bitor(uint32(x11),bitshift(uint32(x12),16)));
    | 
    | end
  function mram_address =MRAM_imu_data_address_actual(cell_no,freq_ind,...:
    | function mram_address =MRAM_imu_data_address_actual(cell_no,freq_ind,...
    | CODE_IMU_DATA)
    | 
    | CODE = uint16([0 0 0 0]);
    | 
    | address_single=single(0);
    | 
    | if CODE_IMU_DATA == IMU_DATA_STORE_REAL
    |     CODE = uint16([hex2dec('02') 0 0 0]);
    |     address_single=(single(cell_no)*(single(NUM_OF_FREQUENCIES)*8))+...
    |         (single(freq_ind)*8)+single(BASIS_ADDRESS_LOCUS);
    | end
    | if CODE_IMU_DATA == IMU_DATA_STORE_IMAG
    |     CODE = uint16([hex2dec('02') 0 0 0]);
    |     address_single=(single(cell_no)*(single(NUM_OF_FREQUENCIES)*8))+...
    |         (single(freq_ind)*8)+4+single(BASIS_ADDRESS_LOCUS);
    | end
    | if CODE_IMU_DATA == IMU_DATA_READ_REAL
    |     CODE = uint16([hex2dec('03') 0 0 0]);
    |    address_single=(single(cell_no)*(single(NUM_OF_FREQUENCIES)*8))+...
    |         (single(freq_ind)*8)+single(BASIS_ADDRESS_LOCUS);
    | end
    | if CODE_IMU_DATA == IMU_DATA_READ_IMAG
    |     CODE = uint16([hex2dec('03') 0 0 0]);
    |    address_single=(single(cell_no)*(single(NUM_OF_FREQUENCIES)*8))+...
    |         (single(freq_ind)*8)+4+single(BASIS_ADDRESS_LOCUS);
    | end
    | 
    | 
    | %address=typecast(address_single,'uint32');
    | address = uint32(address_single);
    | % änderung reihenfolge um adresse richtig für maram zu versenden
    | CODE(4)= uint16(bitand(uint32(hex2dec('000000ff')),address));
    | CODE(3)= uint16(bitand(uint32(hex2dec('000000ff')),bitshift(address,-8)));
    | CODE(2)= uint16(bitand(uint32(hex2dec('000000ff')),bitshift(address,-16)));
    | 
    | 
    | x1=uint16(bitand(uint16(hex2dec('00ff')),uint16(CODE(1))));
    | x2=uint16(bitand(uint16(hex2dec('ff00')),uint16(bitshift(uint16(CODE(2)),8))));
    | x3=uint16(bitand(uint16(hex2dec('00ff')),uint16(CODE(3))));
    | x4=uint16(bitand(uint16(hex2dec('ff00')),uint16(bitshift(uint16(CODE(4)),8))));
    | 
    | x11=uint16(bitor(x1,x2));
    | x12=uint16(bitor(x3,x4));
    | 
    | mram_address=uint32(bitor(uint32(x11),bitshift(uint32(x12),16)));
    | 
    | end
  function mram_address = MRAM_para_address_act(cell_no,para_num,CODE_PARA):
    | function mram_address = MRAM_para_address_act(cell_no,para_num,CODE_PARA)
    | 
    | CODE = uint16([0 0 0 0]);
    | 
    | address_single=single(0);
    | num_of_para = NUM_OF_PARAMETER + single(1);
    | % RS; RD; alpha; k; wg; L2
    | switch CODE_PARA
    |     case PARA_STORE_ACT
    |         CODE = uint16([hex2dec('02') 0 0 0]);
    |         address_single=single(cell_no)*num_of_para*single(4)+...
    |             single(para_num)*single(4)+single(BASIS_ADDRESS_PARA_ACT);
    |     
    |     case PARA_READ_ACT
    |         CODE = uint16([hex2dec('03') 0 0 0]);
    |         address_single=single(cell_no)*num_of_para*single(4)+...
    |             single(para_num)*single(4)+single(BASIS_ADDRESS_PARA_ACT);
    |    
    | end
    | address = uint32(address_single);
    | 
    | % änderung reihenfolge um adresse richtig für maram zu versenden
    | CODE(4)= uint16(bitand(uint32(hex2dec('000000ff')),address));
    | CODE(3)= uint16(bitand(uint32(hex2dec('000000ff')),bitshift(address,-8)));
    | CODE(2)= uint16(bitand(uint32(hex2dec('000000ff')),bitshift(address,-16)));
    | 
    | 
    | x1=uint16(bitand(uint16(hex2dec('00ff')),uint16(CODE(1))));
    | x2=uint16(bitand(uint16(hex2dec('ff00')),uint16(bitshift(uint16(CODE(2)),8))));
    | x3=uint16(bitand(uint16(hex2dec('00ff')),uint16(CODE(3))));
    | x4=uint16(bitand(uint16(hex2dec('ff00')),uint16(bitshift(uint16(CODE(4)),8))));
    | 
    | x11=uint16(bitor(x1,x2));
    | x12=uint16(bitor(x3,x4));
    | 
    | mram_address=uint32(bitor(uint32(x11),bitshift(uint32(x12),16)));
    | 
    | end
  function mram_address = MRAM_address_scc_soc_index(CODE_INDEX):
    | function mram_address = MRAM_address_scc_soc_index(CODE_INDEX)
    | 
    | CODE = uint16([0 0 0 0]);
    | 
    | address_single=single(0);
    | 
    | switch CODE_INDEX
    |     case STORE_LAST_SOC_INDEX
    |         CODE = uint16([hex2dec('02') 0 0 0]);
    |         address_single=single(ADDRESS_LAST_SOC_INDEX);
    |     
    |     case READ_LAST_SOC_INDEX
    |         CODE = uint16([hex2dec('03') 0 0 0]);
    |         address_single=single(ADDRESS_LAST_SOC_INDEX);
    |    
    | end
    | address = uint32(address_single);
    | 
    | % änderung reihenfolge um adresse richtig für maram zu versenden
    | CODE(4)= uint16(bitand(uint32(hex2dec('000000ff')),address));
    | CODE(3)= uint16(bitand(uint32(hex2dec('000000ff')),bitshift(address,-8)));
    | CODE(2)= uint16(bitand(uint32(hex2dec('000000ff')),bitshift(address,-16)));
    | 
    | 
    | x1=uint16(bitand(uint16(hex2dec('00ff')),uint16(CODE(1))));
    | x2=uint16(bitand(uint16(hex2dec('ff00')),uint16(bitshift(uint16(CODE(2)),8))));
    | x3=uint16(bitand(uint16(hex2dec('00ff')),uint16(CODE(3))));
    | x4=uint16(bitand(uint16(hex2dec('ff00')),uint16(bitshift(uint16(CODE(4)),8))));
    | 
    | x11=uint16(bitor(x1,x2));
    | x12=uint16(bitor(x3,x4));
    | 
    | mram_address=uint32(bitor(uint32(x11),bitshift(uint32(x12),16)));
    | 
    | end
  function mram_address = MRAM_para_address_scc(cell_no,para_num,soc_point,CODE_PARA):
    | function mram_address = MRAM_para_address_scc(cell_no,para_num,soc_point,CODE_PARA)
    | 
    | CODE = uint16([0 0 0 0]);
    | 
    | address_single=single(0);
    | num_of_para = NUM_OF_PARAMETER + single(1);
    | % RS; RD; alpha; k; wg; L2
    | switch CODE_PARA
    |     case PARA_STORE_SCC
    |         CODE = uint16([hex2dec('02') 0 0 0]);
    |         address_single = ...
    |             single(cell_no)*num_of_para*single(NUM_OF_SOC_POINTS)*single(4)+...
    |             single(soc_point)*num_of_para*single(4)+...
    |             single(para_num)*single(4)+...
    |             single(BASIS_ADDRESS_PARA_SCC);
    |     case PARA_READ_SCC
    |         CODE = uint16([hex2dec('03') 0 0 0]);
    |         address_single = ...
    |             single(cell_no)*num_of_para*single(NUM_OF_SOC_POINTS)*single(4)+...
    |             single(soc_point)*num_of_para*single(4)+...
    |             single(para_num)*single(4)+...
    |             single(BASIS_ADDRESS_PARA_SCC);
    |     
    |                     
    | end
    | 
    | address = uint32(address_single);
    | % änderung reihenfolge um adresse richtig für maram zu versenden
    | CODE(4)= uint16(bitand(uint32(hex2dec('000000ff')),address));
    | CODE(3)= uint16(bitand(uint32(hex2dec('000000ff')),bitshift(address,-8)));
    | CODE(2)= uint16(bitand(uint32(hex2dec('000000ff')),bitshift(address,-16)));
    | 
    | 
    | x1=uint16(bitand(uint16(hex2dec('00ff')),uint16(CODE(1))));
    | x2=uint16(bitand(uint16(hex2dec('ff00')),uint16(bitshift(uint16(CODE(2)),8))));
    | x3=uint16(bitand(uint16(hex2dec('00ff')),uint16(CODE(3))));
    | x4=uint16(bitand(uint16(hex2dec('ff00')),uint16(bitshift(uint16(CODE(4)),8))));
    | 
    | x11=uint16(bitor(x1,x2));
    | x12=uint16(bitor(x3,x4));
    | 
    | mram_address=uint32(bitor(uint32(x11),bitshift(uint32(x12),16)));
    | 
    | end
  function value_converted = mram_convert_uint32_to_single(value):
    | function value_converted = mram_convert_uint32_to_single(value)
    | % convert uint32 to single representive interger
    | value_converted = typecast(value,'single');
  function value_converted = mram_convert_single_to_uint32(value):
    | function value_converted = mram_convert_single_to_uint32(value)
    | % convert int32 to uint32 representive interger
    | value_converted = typecast(value,'uint32');
  function value_converted = mram_convert_unit32_to_int32(value):
    | function value_converted = mram_convert_unit32_to_int32(value)
    | % convert int32 to uint32 representive interger
    | value_converted = typecast(value,'int32');
  function value = mram_convert_soc(act_soc):
    | function value = mram_convert_soc(act_soc)
    | % convert int32 to uint32 representive interger
    | value = typecast(act_soc,'uint32');
